simulink model "zhengliumoni"  (R2021a)
settings: Solver=VariableStepAuto  StartTime=0.0  StopTime=0.06  RelTol=1e-3
libraries: spsVoltageMeasurementLib x8, spsDetailedThyristorLib x6, spsACVoltageSourceLib x3, spsCurrentMeasurementLib x1, spsDCMachineLib x1, spsDCVoltageSourceLib x1, spsSeriesRLCBranchLib x1, spspowerguiLib x1
settings Model: Creator=HONOR  LastModifiedBy=HONOR

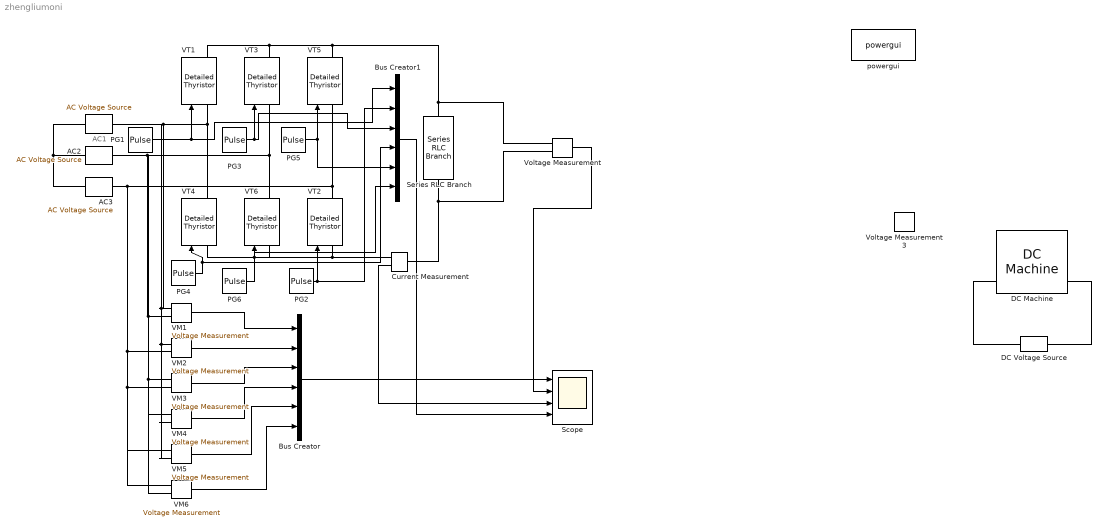
== system zhengliumoni ==
  note: AC1
  " " : spsACVoltageSourceLib/AC Voltage Source  Amplitude=220  Phase=0  Frequency=50  SampleTime=0  Measurements=None  BusType=swing  Pref=10e3  Qref=0  Qmin=-inf  Qmax=+inf
  "AC2 " : spsACVoltageSourceLib/AC Voltage Source  Amplitude=220  Phase=-120  Frequency=50  SampleTime=0  Measurements=None  BusType=swing  Pref=10e3  Qref=0  Qmin=-inf  Qmax=+inf
  AC3 : spsACVoltageSourceLib/AC Voltage Source  Amplitude=220  Phase=-240  Frequency=50  SampleTime=0  Measurements=None  BusType=swing  Pref=10e3  Qref=0  Qmin=-inf  Qmax=+inf
  Bus Creator : BusCreator  Inputs=6
  Bus Creator1 : BusCreator  Inputs=6
  Current Measurement : spsCurrentMeasurementLib/Current Measurement  PhasorSimulation=off  OutputType=Complex  PSBequivalent=0
  DC Machine : spsDCMachineLib/DC Machine  PresetModel=No  MechanicalLoad=Torque TL  FieldType=Wound  ShowDetailedParameters=on  MeasurementBus=off  RLa="[ 0.6  0.012]"  RLf="[ 240  120]"  Laf=1.8  MachineConstant=Torque constant (N.m/A)  Ke=1.8  Kt=1.8  J=1  Bm=0  Tf=0  w0=1  Ifinit=0.416666666255433  TsPowergui=0  TsBlock=-1
  DC Voltage Source : spsDCVoltageSourceLib/DC Voltage Source  Amplitude=100  Measurements=None
  PG1 : DiscretePulseGenerator  PulseType=Time based  Period=0.02  PulseWidth=20  PhaseDelay=0.0067
  PG2 : DiscretePulseGenerator  PulseType=Time based  Period=0.02  PulseWidth=20  PhaseDelay=0.01
  PG3 : DiscretePulseGenerator  PulseType=Time based  Period=0.02  PulseWidth=20  PhaseDelay=0.0133
  PG4 : DiscretePulseGenerator  PulseType=Time based  Period=0.02  PulseWidth=20  PhaseDelay=0.0167
  PG5 : DiscretePulseGenerator  PulseType=Time based  Period=0.02  PulseWidth=20  PhaseDelay=0.02
  PG6 : DiscretePulseGenerator  PulseType=Time based  Period=0.02  PulseWidth=20  PhaseDelay=0.0233
  Scope : Scope  NumInputPorts=4
  Series RLC Branch : spsSeriesRLCBranchLib/Series RLC Branch  LConnTagsString=__new0  RConnTagsString=__new0  BranchType=RL  Resistance=10  Inductance=10  SetiL0=off  InitialCurrent=0  Capacitance=1e-6  Setx0=off  InitialVoltage=0  Measurements=None
  VM{1..6} (6 alike) : spsVoltageMeasurementLib/Voltage Measurement  PhasorSimulation=off  OutputType=Complex  PSBequivalent=0
  "VT1 " : spsDetailedThyristorLib/Detailed Thyristor  Ron=0.001  Lon=1e-3  Vf=0.8  IL=0.1  Tq=100e-6  IC=0  Rs=500  Cs=250e-9  Measurements=on
      settings: SourceProductBaseCode=PS
  VT{2..6} (5 alike) : spsDetailedThyristorLib/Detailed Thyristor  Ron=0.001  Lon=1e-3  Vf=0.8  IL=0.1  Tq=100e-6  IC=0  Rs=500  Cs=250e-9  Measurements=on
      settings: SourceProductBaseCode=PS
  Voltage Measurement : spsVoltageMeasurementLib/Voltage Measurement  PhasorSimulation=off  OutputType=Complex  PSBequivalent=0
  Voltage Measurement3 : spsVoltageMeasurementLib/Voltage Measurement  PhasorSimulation=off  OutputType=Complex  PSBequivalent=0
  powergui : spspowerguiLib/powergui  Priority=1  SimulationMode=Continuous  SampleTime=50e-6  frequency=60  Iterations=50  frequencyindice=0  Pbase=100e6  ErrMax=1e-4  UnitsV=kV  UnitsW=MW  buscounter=0  FunctionMessages=off  echomessages=off  EnableUseOfTLC=off  CurrentSourceSwitches=off  DisableSnubberDevices=off  DisableRonSwitches=off  DisableVfSwitches=off  DisplayEquations=off  AutomaticDiscreteSolvers=off  SolverType=Tustin/Backward Euler (TBE)  Interpol=off  ExternalGateDelay=off  methode=off  Ts=100  x0status=blocks  SPID=on  SwTol=0  HookPort=off  NonlinearTolerance=1e-4  nMaxIteration=100  ContinueOnMaxIteration=off  RestoreLinks=warning  ResistiveCurrentMeasurement=off  Frange=[0:2:500]  Ylog=off  Xlog=on  ShowGrid=off  save=off  variable=ZData  structure=0  ZoomFFT=off  StartTime=0.0  cycles=1  DisplayStyle=1  fundamental=60  FreqAxis=off  MaxFrequency=1000  frequencyindicesteady=1  RmsSteady=1  display=off
  wires:
  VM1/1 -> Bus Creator/1
  VM2/1 -> Bus Creator/2
  VM3/1 -> Bus Creator/3
  VM4/1 -> Bus Creator/4
  VM5/1 -> Bus Creator/5
  VM6/1 -> Bus Creator/6
  Bus Creator/1 -> Scope/1
  PG4/1 -> Bus Creator1/4, VT4/1
  PG6/1 -> Bus Creator1/6, VT6/1
  PG5/1 -> Bus Creator1/5, VT5/1
  Voltage Measurement/1 -> Scope/2
  Current Measurement/1 -> Scope/3
  Bus Creator1/1 -> Scope/4
  PG1/1 -> "VT1 "/1, Bus Creator1/1
  PG2/1 -> VT2/1, Bus Creator1/2
  PG3/1 -> VT3/1, Bus Creator1/3
  connections:
  VT5/LConn1 -- VM6/LConn1 -- VM5/LConn1 -- VM3/LConn2 -- VM2/LConn2 -- AC3/RConn1 -- VT2/RConn1
  VT3/LConn1 -- VM6/LConn2 -- VM4/LConn1 -- VM3/LConn1 -- VM1/LConn2 -- "AC2 "/RConn1 -- VT6/RConn1
  "VT1 "/LConn1 -- VM5/LConn2 -- VM4/LConn2 -- VM2/LConn1 -- VM1/LConn1 -- " "/RConn1 -- VT4/RConn1
  Current Measurement/LConn1 -- Series RLC Branch/RConn1 -- Voltage Measurement/LConn2
  Current Measurement/RConn1 -- VT4/LConn1 -- VT6/LConn1 -- VT2/LConn1
  Series RLC Branch/LConn1 -- Voltage Measurement/LConn1 -- VT5/RConn1 -- VT3/RConn1 -- "VT1 "/RConn1
  AC3/LConn1 -- " "/LConn1 -- "AC2 "/LConn1
  DC Machine/RConn2 -- DC Voltage Source/LConn1
  DC Voltage Source/RConn1 -- DC Machine/LConn2
